simulink library "rvs"  (R2016a)
settings: Solver=ode45  StartTime=0.0  StopTime=10.0  RelTol=1e-3
settings Model: Creator=Arthur  LastModifiedBy=aeagr
settings DataIOCC: LimitDataPoints=on  SaveFormat=Array
settings DebuggingCC: SolverPrmCheckMsg=warning
settings HardwareCC: ProdBitPerPointer=32  ProdLargestAtomicFloat=None  ProdIntDivRoundTo=Undefined  ProdEndianess=Unspecified  ProdWordSize=32  ProdHWDeviceType=32-bit Generic
settings ModelReferenceCC: PropagateSignalLabelsOutOfModel=off
settings ConfigComp: CovModelRefEnable=Off  CovSFcnEnable=off

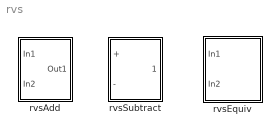
== system rvs ==
  rvsAdd : Subsystem  TreatAsAtomicUnit=on  mask(rvsAdd){}
      mask help: Add two signals
  rvsEquiv : Subsystem  TreatAsAtomicUnit=on  mask(rvsEquiv){}
      mask help: Test equivalence between two input signals.
  rvsSubtract : Subsystem  TreatAsAtomicUnit=on  mask(rvsSubtract){}
      mask help: Subtract two signals

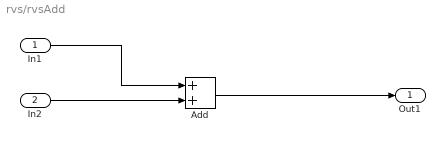
== system rvs/rvsAdd ==
  In1 : Inport
  In2 : Inport  Port=2
  Add : Sum
  Out1 : Outport
  wires:
  Add/1 -> Out1/1
  In2/1 -> Add/2
  In1/1 -> Add/1

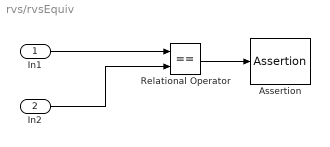
== system rvs/rvsEquiv ==
  In1 : Inport
  In2 : Inport  Port=2
  Assertion : Assertion
  Relational Operator : RelationalOperator  Operator===  OutDataTypeStr=boolean
  wires:
  In1/1 -> Relational Operator/1
  In2/1 -> Relational Operator/2
  Relational Operator/1 -> Assertion/1

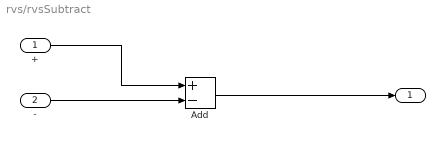
== system rvs/rvsSubtract ==
  + : Inport
  - : Inport  Port=2
  Add : Sum  Inputs=+-
  " " : Outport
  wires:
  Add/1 -> " "/1
  -/1 -> Add/2
  +/1 -> Add/1
